simulink model "SimiSnake5"  (R2019a)
settings: Solver=VariableStepAuto  StartTime=0.0  StopTime=20  RelTol=1e-3  EnableMultiTasking=on
PreLoadFcn:
  | robotParameters;
undefined symbols (not defined in the file or in its folder): X, Y, Z
libraries: nesl_utility x49, sm_lib x38
(part 2 of 2)

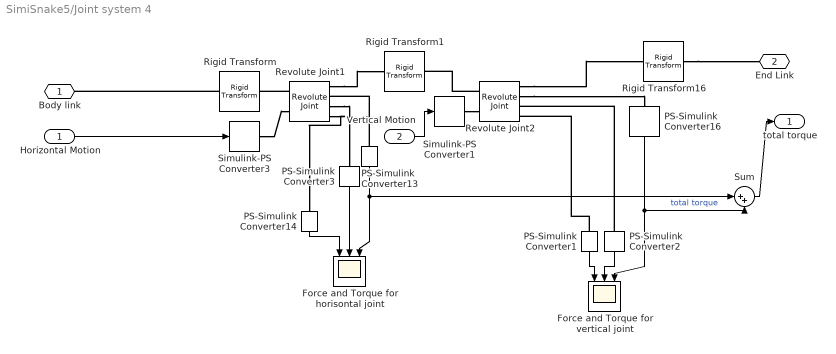
== system SimiSnake5/Joint system 4 ==
  Horizontal Motion : Inport
  Vertical Motion : Inport  Port=2
  Force and Torque for horisontal joint : Scope  NumInputPorts=3
  Force and Torque for vertical joint : Scope  NumInputPorts=3
  PS-Simulink Converter{1,13..14,16} (4 alike) : nesl_utility/PS-Simulink Converter  PhysicalDomain=network_engine_domain  SubClassName=ps_output  LeftPortType=input  RightPortType=output  PseudoPeriodic=off  Frequencies=[]  Unit=N*m  AffineConversion=off
  PS-Simulink Converter2 : nesl_utility/PS-Simulink Converter  PhysicalDomain=network_engine_domain  SubClassName=ps_output  LeftPortType=input  RightPortType=output  PseudoPeriodic=off  Frequencies=[]  Unit=N  AffineConversion=off
  PS-Simulink Converter3 : nesl_utility/PS-Simulink Converter  PhysicalDomain=network_engine_domain  SubClassName=ps_output  LeftPortType=input  RightPortType=output  PseudoPeriodic=off  Frequencies=[]  Unit=N  AffineConversion=off
  Revolute Joint1 : sm_lib/Joints/Revolute Joint  SenseConstraintForce=off  SenseConstraintForceX=off  SenseConstraintForceY=off  SenseConstraintForceZ=off  SenseConstraintTorque=off  SenseConstraintTorqueX=off  SenseConstraintTorqueY=off  SenseConstraintTorqueZ=off  SenseTotalForce=on  SenseTotalForceX=off  SenseTotalForceY=off  SenseTotalForceZ=off  SenseTotalTorque=on  SenseTotalTorqueX=off  SenseTotalTorqueY=off  SenseTotalTorqueZ=off  CompositeWrenchDir=FollowerOnBase  CompositeWrenchFrame=BaseFrame  EquilibriumPosition=0  EquilibriumPositionUnits=deg  SpringStiffness=0  SpringStiffnessUnits=N*m/deg  DampingCoefficient=0  DampingCoefficientUnits=N*m/(deg/s)  TorqueActuationMode=ComputedTorque  MotionActuationMode=InputMotion  SensePosition=off  SenseVelocity=off  SenseAcceleration=off  SenseTorqueForce=on  SenseLowerLimitTorqueForce=off  SenseUpperLimitTorqueForce=off  LowerLimitSpecify=off  LowerLimitBound=-90  LowerLimitBoundUnits=deg  LowerLimitStiffness=1e4  LowerLimitStiffnessUnits=N*m/deg  LowerLimitDamping=10  LowerLimitDampingUnits=N*m/(deg/s)  LowerLimitTransitionRegionWidth=0.1  LowerLimitTransitionRegionWidthUnits=deg  UpperLimitSpecify=off  UpperLimitBound=90  UpperLimitBoundUnits=deg  UpperLimitStiffness=1e4  UpperLimitStiffnessUnits=N*m/deg  UpperLimitDamping=10  UpperLimitDampingUnits=N*m/(deg/s)  UpperLimitTransitionRegionWidth=0.1  UpperLimitTransitionRegionWidthUnits=deg  PositionTargetSpecify=off  PositionTargetPriority=High  PositionTargetValue=30  PositionTargetValueUnits=deg  VelocityTargetSpecify=off  VelocityTargetPriority=High  VelocityTargetValue=0  VelocityTargetValueUnits=deg/s
  Revolute Joint2 : sm_lib/Joints/Revolute Joint  SenseConstraintForce=off  SenseConstraintForceX=off  SenseConstraintForceY=off  SenseConstraintForceZ=off  SenseConstraintTorque=off  SenseConstraintTorqueX=off  SenseConstraintTorqueY=off  SenseConstraintTorqueZ=off  SenseTotalForce=on  SenseTotalForceX=off  SenseTotalForceY=off  SenseTotalForceZ=off  SenseTotalTorque=on  SenseTotalTorqueX=off  SenseTotalTorqueY=off  SenseTotalTorqueZ=off  CompositeWrenchDir=FollowerOnBase  CompositeWrenchFrame=BaseFrame  EquilibriumPosition=0  EquilibriumPositionUnits=deg  SpringStiffness=0  SpringStiffnessUnits=N*m/deg  DampingCoefficient=0  DampingCoefficientUnits=N*m/(deg/s)  TorqueActuationMode=ComputedTorque  MotionActuationMode=InputMotion  SensePosition=off  SenseVelocity=off  SenseAcceleration=off  SenseTorqueForce=on  SenseLowerLimitTorqueForce=off  SenseUpperLimitTorqueForce=off  LowerLimitSpecify=off  LowerLimitBound=-90  LowerLimitBoundUnits=deg  LowerLimitStiffness=1e4  LowerLimitStiffnessUnits=N*m/deg  LowerLimitDamping=10  LowerLimitDampingUnits=N*m/(deg/s)  LowerLimitTransitionRegionWidth=0.1  LowerLimitTransitionRegionWidthUnits=deg  UpperLimitSpecify=off  UpperLimitBound=90  UpperLimitBoundUnits=deg  UpperLimitStiffness=1e4  UpperLimitStiffnessUnits=N*m/deg  UpperLimitDamping=10  UpperLimitDampingUnits=N*m/(deg/s)  UpperLimitTransitionRegionWidth=0.1  UpperLimitTransitionRegionWidthUnits=deg  PositionTargetSpecify=off  PositionTargetPriority=High  PositionTargetValue=30  PositionTargetValueUnits=deg  VelocityTargetSpecify=off  VelocityTargetPriority=High  VelocityTargetValue=0  VelocityTargetValueUnits=deg/s
  Rigid Transform : sm_lib/Frames and Transforms/Rigid Transform  TranslationMethod=StandardAxis  TranslationStandardOffset=5  TranslationLengthUnit=cm  TranslationStandardAxis=-Z  TranslationCartesianOffset=[0 0 0]  TranslationROffset=0  TranslationROffsetUnits=m  TranslationZOffset=0  TranslationZOffsetUnits=m  TranslationThetaOffset=0  TranslationThetaOffsetUnits=deg  RotationMethod=StandardAxis  RotationAngleUnits=deg  RotationStandardAxis=+X  RotationAngle=90  RotationArbitraryAxis=[0 0 1]  FollAlignAxisA=+X  BaseAlignAxisA=+Y  FollAlignAxisB=+Y  BaseAlignAxisB=+Z  RotationSequenceAxes=FollowerAxes  RotationSequence=XYX  RotationSequenceAngles=[0 0 0]  RotationSequenceAnglesUnits=deg  RotationMatrix=[1 0 0; 0 1 0; 0 0 1]
  Rigid Transform1 : sm_lib/Frames and Transforms/Rigid Transform  TranslationMethod=None  TranslationStandardOffset=5  TranslationLengthUnit=cm  TranslationStandardAxis=-Z  TranslationCartesianOffset=[0 0 0]  TranslationROffset=0  TranslationROffsetUnits=m  TranslationZOffset=0  TranslationZOffsetUnits=m  TranslationThetaOffset=0  TranslationThetaOffsetUnits=deg  RotationMethod=StandardAxis  RotationAngleUnits=deg  RotationStandardAxis=+X  RotationAngle=90  RotationArbitraryAxis=[0 0 1]  FollAlignAxisA=+X  BaseAlignAxisA=+Y  FollAlignAxisB=+Y  BaseAlignAxisB=+Z  RotationSequenceAxes=FollowerAxes  RotationSequence=XYX  RotationSequenceAngles=[0 0 0]  RotationSequenceAnglesUnits=deg  RotationMatrix=[1 0 0; 0 1 0; 0 0 1]
  Rigid Transform16 : sm_lib/Frames and Transforms/Rigid Transform  TranslationMethod=StandardAxis  TranslationStandardOffset=5  TranslationLengthUnit=cm  TranslationStandardAxis=+Z  TranslationCartesianOffset=[0 0 0]  TranslationROffset=0  TranslationROffsetUnits=m  TranslationZOffset=0  TranslationZOffsetUnits=m  TranslationThetaOffset=0  TranslationThetaOffsetUnits=deg  RotationMethod=StandardAxis  RotationAngleUnits=deg  RotationStandardAxis=-X  RotationAngle=180  RotationArbitraryAxis=[0 0 1]  FollAlignAxisA=+X  BaseAlignAxisA=+Y  FollAlignAxisB=+Y  BaseAlignAxisB=+Z  RotationSequenceAxes=FollowerAxes  RotationSequence=XYX  RotationSequenceAngles=[0 0 0]  RotationSequenceAnglesUnits=deg  RotationMatrix=[1 0 0; 0 1 0; 0 0 1]
  Simulink-PS Converter1 : nesl_utility/Simulink-PS Converter  PhysicalDomain=network_engine_domain  SubClassName=ps_input  LeftPortType=input  RightPortType=output  PseudoPeriodic=off  Frequencies=[]  NoiseDistribution=none  NoiseParameters=[]  Unit=deg  AffineConversion=off  FilteringAndDerivatives=filter  SimscapeFilterOrder=2  InputFilterTimeConstant=.01  UdotUserProvided=1
  Simulink-PS Converter3 : nesl_utility/Simulink-PS Converter  PhysicalDomain=network_engine_domain  SubClassName=ps_input  LeftPortType=input  RightPortType=output  PseudoPeriodic=off  Frequencies=[]  NoiseDistribution=none  NoiseParameters=[]  Unit=deg  AffineConversion=off  FilteringAndDerivatives=filter  SimscapeFilterOrder=2  InputFilterTimeConstant=.01  UdotUserProvided=1
  Sum : Sum  Inputs=|++
  Body link : PMIOPort  Side=Left
  "End Link " : PMIOPort  Port=2  Side=Right
  total torque : Outport
  wires:
  Vertical Motion/1 -> Simulink-PS Converter1/1
  PS-Simulink Converter14/1 -> Force and Torque for horisontal joint/1
  PS-Simulink Converter13/1 -> Force and Torque for horisontal joint/3, Sum/1
  PS-Simulink Converter3/1 -> Force and Torque for horisontal joint/2
  Horizontal Motion/1 -> Simulink-PS Converter3/1
  PS-Simulink Converter2/1 -> Force and Torque for vertical joint/2
  PS-Simulink Converter1/1 -> Force and Torque for vertical joint/1
  Sum/1 -> total torque/1
  PS-Simulink Converter16/1 -> Force and Torque for vertical joint/3, Sum/2  "total torque"
  connections:
  Simulink-PS Converter3/RConn1 -- Revolute Joint1/LConn2
  Revolute Joint1/RConn1 -- Rigid Transform1/LConn1
  Rigid Transform/LConn1 -- Body link/RConn1
  Revolute Joint1/RConn4 -- PS-Simulink Converter14/LConn1
  Revolute Joint1/RConn3 -- PS-Simulink Converter3/LConn1
  Revolute Joint2/RConn2 -- PS-Simulink Converter16/LConn1
  Revolute Joint2/RConn1 -- Rigid Transform16/LConn1
  PS-Simulink Converter13/LConn1 -- Revolute Joint1/RConn2
  Revolute Joint1/LConn1 -- Rigid Transform/RConn1
  Simulink-PS Converter1/RConn1 -- Revolute Joint2/LConn2
  Revolute Joint2/LConn1 -- Rigid Transform1/RConn1
  PS-Simulink Converter2/LConn1 -- Revolute Joint2/RConn3
  PS-Simulink Converter1/LConn1 -- Revolute Joint2/RConn4
  Rigid Transform16/RConn1 -- "End Link "/RConn1

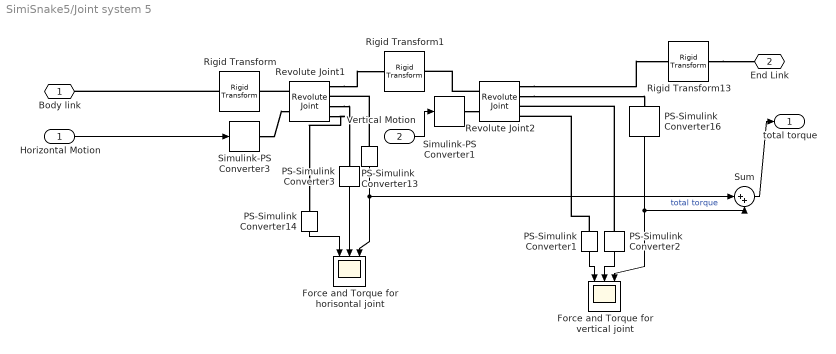
== system SimiSnake5/Joint system 5 ==
  Horizontal Motion : Inport
  Vertical Motion : Inport  Port=2
  Force and Torque for horisontal joint : Scope  NumInputPorts=3
  Force and Torque for vertical joint : Scope  NumInputPorts=3
  PS-Simulink Converter{1,13..14,16} (4 alike) : nesl_utility/PS-Simulink Converter  PhysicalDomain=network_engine_domain  SubClassName=ps_output  LeftPortType=input  RightPortType=output  PseudoPeriodic=off  Frequencies=[]  Unit=N*m  AffineConversion=off
  PS-Simulink Converter2 : nesl_utility/PS-Simulink Converter  PhysicalDomain=network_engine_domain  SubClassName=ps_output  LeftPortType=input  RightPortType=output  PseudoPeriodic=off  Frequencies=[]  Unit=N  AffineConversion=off
  PS-Simulink Converter3 : nesl_utility/PS-Simulink Converter  PhysicalDomain=network_engine_domain  SubClassName=ps_output  LeftPortType=input  RightPortType=output  PseudoPeriodic=off  Frequencies=[]  Unit=N  AffineConversion=off
  Revolute Joint1 : sm_lib/Joints/Revolute Joint  SenseConstraintForce=off  SenseConstraintForceX=off  SenseConstraintForceY=off  SenseConstraintForceZ=off  SenseConstraintTorque=off  SenseConstraintTorqueX=off  SenseConstraintTorqueY=off  SenseConstraintTorqueZ=off  SenseTotalForce=on  SenseTotalForceX=off  SenseTotalForceY=off  SenseTotalForceZ=off  SenseTotalTorque=on  SenseTotalTorqueX=off  SenseTotalTorqueY=off  SenseTotalTorqueZ=off  CompositeWrenchDir=FollowerOnBase  CompositeWrenchFrame=BaseFrame  EquilibriumPosition=0  EquilibriumPositionUnits=deg  SpringStiffness=0  SpringStiffnessUnits=N*m/deg  DampingCoefficient=0  DampingCoefficientUnits=N*m/(deg/s)  TorqueActuationMode=ComputedTorque  MotionActuationMode=InputMotion  SensePosition=off  SenseVelocity=off  SenseAcceleration=off  SenseTorqueForce=on  SenseLowerLimitTorqueForce=off  SenseUpperLimitTorqueForce=off  LowerLimitSpecify=off  LowerLimitBound=-90  LowerLimitBoundUnits=deg  LowerLimitStiffness=1e4  LowerLimitStiffnessUnits=N*m/deg  LowerLimitDamping=10  LowerLimitDampingUnits=N*m/(deg/s)  LowerLimitTransitionRegionWidth=0.1  LowerLimitTransitionRegionWidthUnits=deg  UpperLimitSpecify=off  UpperLimitBound=90  UpperLimitBoundUnits=deg  UpperLimitStiffness=1e4  UpperLimitStiffnessUnits=N*m/deg  UpperLimitDamping=10  UpperLimitDampingUnits=N*m/(deg/s)  UpperLimitTransitionRegionWidth=0.1  UpperLimitTransitionRegionWidthUnits=deg  PositionTargetSpecify=off  PositionTargetPriority=High  PositionTargetValue=30  PositionTargetValueUnits=deg  VelocityTargetSpecify=off  VelocityTargetPriority=High  VelocityTargetValue=0  VelocityTargetValueUnits=deg/s
  Revolute Joint2 : sm_lib/Joints/Revolute Joint  SenseConstraintForce=off  SenseConstraintForceX=off  SenseConstraintForceY=off  SenseConstraintForceZ=off  SenseConstraintTorque=off  SenseConstraintTorqueX=off  SenseConstraintTorqueY=off  SenseConstraintTorqueZ=off  SenseTotalForce=on  SenseTotalForceX=off  SenseTotalForceY=off  SenseTotalForceZ=off  SenseTotalTorque=on  SenseTotalTorqueX=off  SenseTotalTorqueY=off  SenseTotalTorqueZ=off  CompositeWrenchDir=FollowerOnBase  CompositeWrenchFrame=BaseFrame  EquilibriumPosition=0  EquilibriumPositionUnits=deg  SpringStiffness=0  SpringStiffnessUnits=N*m/deg  DampingCoefficient=0  DampingCoefficientUnits=N*m/(deg/s)  TorqueActuationMode=ComputedTorque  MotionActuationMode=InputMotion  SensePosition=off  SenseVelocity=off  SenseAcceleration=off  SenseTorqueForce=on  SenseLowerLimitTorqueForce=off  SenseUpperLimitTorqueForce=off  LowerLimitSpecify=off  LowerLimitBound=-90  LowerLimitBoundUnits=deg  LowerLimitStiffness=1e4  LowerLimitStiffnessUnits=N*m/deg  LowerLimitDamping=10  LowerLimitDampingUnits=N*m/(deg/s)  LowerLimitTransitionRegionWidth=0.1  LowerLimitTransitionRegionWidthUnits=deg  UpperLimitSpecify=off  UpperLimitBound=90  UpperLimitBoundUnits=deg  UpperLimitStiffness=1e4  UpperLimitStiffnessUnits=N*m/deg  UpperLimitDamping=10  UpperLimitDampingUnits=N*m/(deg/s)  UpperLimitTransitionRegionWidth=0.1  UpperLimitTransitionRegionWidthUnits=deg  PositionTargetSpecify=off  PositionTargetPriority=High  PositionTargetValue=30  PositionTargetValueUnits=deg  VelocityTargetSpecify=off  VelocityTargetPriority=High  VelocityTargetValue=0  VelocityTargetValueUnits=deg/s
  Rigid Transform : sm_lib/Frames and Transforms/Rigid Transform  TranslationMethod=StandardAxis  TranslationStandardOffset=5  TranslationLengthUnit=cm  TranslationStandardAxis=-Z  TranslationCartesianOffset=[0 0 0]  TranslationROffset=0  TranslationROffsetUnits=m  TranslationZOffset=0  TranslationZOffsetUnits=m  TranslationThetaOffset=0  TranslationThetaOffsetUnits=deg  RotationMethod=StandardAxis  RotationAngleUnits=deg  RotationStandardAxis=+X  RotationAngle=90  RotationArbitraryAxis=[0 0 1]  FollAlignAxisA=+X  BaseAlignAxisA=+Y  FollAlignAxisB=+Y  BaseAlignAxisB=+Z  RotationSequenceAxes=FollowerAxes  RotationSequence=XYX  RotationSequenceAngles=[0 0 0]  RotationSequenceAnglesUnits=deg  RotationMatrix=[1 0 0; 0 1 0; 0 0 1]
  Rigid Transform1 : sm_lib/Frames and Transforms/Rigid Transform  TranslationMethod=None  TranslationStandardOffset=5  TranslationLengthUnit=cm  TranslationStandardAxis=-Z  TranslationCartesianOffset=[0 0 0]  TranslationROffset=0  TranslationROffsetUnits=m  TranslationZOffset=0  TranslationZOffsetUnits=m  TranslationThetaOffset=0  TranslationThetaOffsetUnits=deg  RotationMethod=StandardAxis  RotationAngleUnits=deg  RotationStandardAxis=+X  RotationAngle=90  RotationArbitraryAxis=[0 0 1]  FollAlignAxisA=+X  BaseAlignAxisA=+Y  FollAlignAxisB=+Y  BaseAlignAxisB=+Z  RotationSequenceAxes=FollowerAxes  RotationSequence=XYX  RotationSequenceAngles=[0 0 0]  RotationSequenceAnglesUnits=deg  RotationMatrix=[1 0 0; 0 1 0; 0 0 1]
  Rigid Transform13 : sm_lib/Frames and Transforms/Rigid Transform  TranslationMethod=StandardAxis  TranslationStandardOffset=5  TranslationLengthUnit=cm  TranslationStandardAxis=+Z  TranslationCartesianOffset=[0 0 0]  TranslationROffset=0  TranslationROffsetUnits=m  TranslationZOffset=0  TranslationZOffsetUnits=m  TranslationThetaOffset=0  TranslationThetaOffsetUnits=deg  RotationMethod=StandardAxis  RotationAngleUnits=deg  RotationStandardAxis=-X  RotationAngle=180  RotationArbitraryAxis=[0 0 1]  FollAlignAxisA=+X  BaseAlignAxisA=+Y  FollAlignAxisB=+Y  BaseAlignAxisB=+Z  RotationSequenceAxes=FollowerAxes  RotationSequence=XYX  RotationSequenceAngles=[0 0 0]  RotationSequenceAnglesUnits=deg  RotationMatrix=[1 0 0; 0 1 0; 0 0 1]
  Simulink-PS Converter1 : nesl_utility/Simulink-PS Converter  PhysicalDomain=network_engine_domain  SubClassName=ps_input  LeftPortType=input  RightPortType=output  PseudoPeriodic=off  Frequencies=[]  NoiseDistribution=none  NoiseParameters=[]  Unit=deg  AffineConversion=off  FilteringAndDerivatives=filter  SimscapeFilterOrder=2  InputFilterTimeConstant=.01  UdotUserProvided=1
  Simulink-PS Converter3 : nesl_utility/Simulink-PS Converter  PhysicalDomain=network_engine_domain  SubClassName=ps_input  LeftPortType=input  RightPortType=output  PseudoPeriodic=off  Frequencies=[]  NoiseDistribution=none  NoiseParameters=[]  Unit=deg  AffineConversion=off  FilteringAndDerivatives=filter  SimscapeFilterOrder=2  InputFilterTimeConstant=.01  UdotUserProvided=1
  Sum : Sum  Inputs=|++
  Body link : PMIOPort  Side=Left
  "End Link " : PMIOPort  Port=2  Side=Right
  total torque : Outport
  wires:
  Vertical Motion/1 -> Simulink-PS Converter1/1
  PS-Simulink Converter14/1 -> Force and Torque for horisontal joint/1
  PS-Simulink Converter13/1 -> Force and Torque for horisontal joint/3, Sum/1
  PS-Simulink Converter3/1 -> Force and Torque for horisontal joint/2
  Horizontal Motion/1 -> Simulink-PS Converter3/1
  PS-Simulink Converter2/1 -> Force and Torque for vertical joint/2
  PS-Simulink Converter1/1 -> Force and Torque for vertical joint/1
  Sum/1 -> total torque/1
  PS-Simulink Converter16/1 -> Force and Torque for vertical joint/3, Sum/2  "total torque"
  connections:
  Simulink-PS Converter3/RConn1 -- Revolute Joint1/LConn2
  Revolute Joint1/RConn1 -- Rigid Transform1/LConn1
  Rigid Transform/LConn1 -- Body link/RConn1
  Revolute Joint1/RConn4 -- PS-Simulink Converter14/LConn1
  Revolute Joint1/RConn3 -- PS-Simulink Converter3/LConn1
  Revolute Joint2/RConn2 -- PS-Simulink Converter16/LConn1
  Rigid Transform13/RConn1 -- "End Link "/RConn1
  PS-Simulink Converter13/LConn1 -- Revolute Joint1/RConn2
  Revolute Joint1/LConn1 -- Rigid Transform/RConn1
  Simulink-PS Converter1/RConn1 -- Revolute Joint2/LConn2
  Revolute Joint2/LConn1 -- Rigid Transform1/RConn1
  PS-Simulink Converter2/LConn1 -- Revolute Joint2/RConn3
  PS-Simulink Converter1/LConn1 -- Revolute Joint2/RConn4
  Revolute Joint2/RConn1 -- Rigid Transform13/LConn1

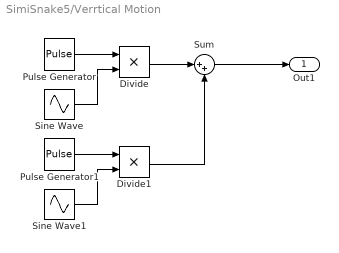
== system SimiSnake5/Verrtical Motion  ==
  Divide : Product  Inputs=**
  Divide1 : Product  Inputs=**
  Pulse Generator : DiscretePulseGenerator  PulseType=Time based  PulseWidth=50
  Pulse Generator1 : DiscretePulseGenerator  PulseType=Time based  PulseWidth=50  PhaseDelay=1
  Sine Wave : Sin  Amplitude=20  Frequency=5  Phase=2.09
  Sine Wave1 : Sin  Amplitude=15  Frequency=5  Phase=2.09
  Sum : Sum  Inputs=|++
  Out1 : Outport
  wires:
  Sum/1 -> Out1/1
  Divide1/1 -> Sum/2
  Divide/1 -> Sum/1
  Pulse Generator/1 -> Divide/1
  Sine Wave1/1 -> Divide1/2
  Sine Wave/1 -> Divide/2
  Pulse Generator1/1 -> Divide1/1

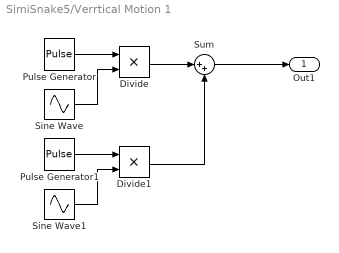
== system SimiSnake5/Verrtical Motion 1 ==
  Divide : Product  Inputs=**
  Divide1 : Product  Inputs=**
  Pulse Generator : DiscretePulseGenerator  PulseType=Time based  PulseWidth=50
  Pulse Generator1 : DiscretePulseGenerator  PulseType=Time based  PulseWidth=50  PhaseDelay=1
  Sine Wave : Sin  Amplitude=20  Frequency=5  Phase=2 * 2.09  SampleTime=0
  Sine Wave1 : Sin  Amplitude=15  Frequency=5  Phase=2.09 * 2  SampleTime=0
  Sum : Sum  Inputs=|++
  Out1 : Outport
  wires:
  Sum/1 -> Out1/1
  Divide1/1 -> Sum/2
  Divide/1 -> Sum/1
  Pulse Generator/1 -> Divide/1
  Sine Wave1/1 -> Divide1/2
  Sine Wave/1 -> Divide/2
  Pulse Generator1/1 -> Divide1/1

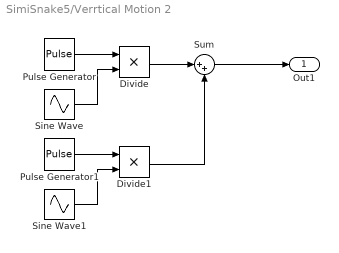
== system SimiSnake5/Verrtical Motion 2 ==
  Divide : Product  Inputs=**
  Divide1 : Product  Inputs=**
  Pulse Generator : DiscretePulseGenerator  PulseType=Time based  PulseWidth=50
  Pulse Generator1 : DiscretePulseGenerator  PulseType=Time based  PulseWidth=50  PhaseDelay=1
  Sine Wave : Sin  Amplitude=20  Frequency=5  Phase=2.09 * 3  SampleTime=0
  Sine Wave1 : Sin  Amplitude=15  Frequency=5  Phase=2.09 * 3  SampleTime=0
  Sum : Sum  Inputs=|++
  Out1 : Outport
  wires:
  Sum/1 -> Out1/1
  Divide1/1 -> Sum/2
  Divide/1 -> Sum/1
  Pulse Generator/1 -> Divide/1
  Sine Wave1/1 -> Divide1/2
  Sine Wave/1 -> Divide/2
  Pulse Generator1/1 -> Divide1/1

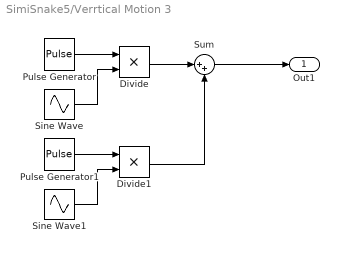
== system SimiSnake5/Verrtical Motion 3 ==
  Divide : Product  Inputs=**
  Divide1 : Product  Inputs=**
  Pulse Generator : DiscretePulseGenerator  PulseType=Time based  PulseWidth=50
  Pulse Generator1 : DiscretePulseGenerator  PulseType=Time based  PulseWidth=50  PhaseDelay=1
  Sine Wave : Sin  Amplitude=20  Frequency=5  Phase=2.09 * 4  SampleTime=0
  Sine Wave1 : Sin  Amplitude=15  Frequency=5  Phase=2.09 * 4  SampleTime=0
  Sum : Sum  Inputs=|++
  Out1 : Outport
  wires:
  Sum/1 -> Out1/1
  Divide1/1 -> Sum/2
  Divide/1 -> Sum/1
  Pulse Generator/1 -> Divide/1
  Sine Wave1/1 -> Divide1/2
  Sine Wave/1 -> Divide/2
  Pulse Generator1/1 -> Divide1/1

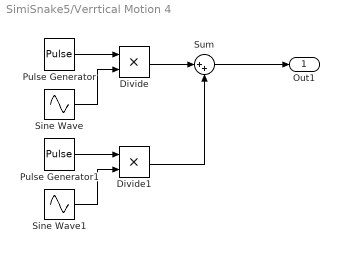
== system SimiSnake5/Verrtical Motion 4 ==
  Divide : Product  Inputs=**
  Divide1 : Product  Inputs=**
  Pulse Generator : DiscretePulseGenerator  PulseType=Time based  PulseWidth=50
  Pulse Generator1 : DiscretePulseGenerator  PulseType=Time based  PulseWidth=50  PhaseDelay=1
  Sine Wave : Sin  Amplitude=20  Frequency=5  Phase=2.09 * 5  SampleTime=0
  Sine Wave1 : Sin  Amplitude=15  Frequency=5  Phase=2.09 * 5  SampleTime=0
  Sum : Sum  Inputs=|++
  Out1 : Outport
  wires:
  Sum/1 -> Out1/1
  Divide1/1 -> Sum/2
  Divide/1 -> Sum/1
  Pulse Generator/1 -> Divide/1
  Sine Wave1/1 -> Divide1/2
  Sine Wave/1 -> Divide/2
  Pulse Generator1/1 -> Divide1/1

== system SimiSnake5/Verrtical Motion 5 ==
  Divide : Product  Inputs=**
  Divide1 : Product  Inputs=**
  Pulse Generator : DiscretePulseGenerator  PulseType=Time based  PulseWidth=50
  Pulse Generator1 : DiscretePulseGenerator  PulseType=Time based  PulseWidth=50  PhaseDelay=1
  Sine Wave : Sin  Amplitude=20  Frequency=5  Phase=2.09 * 6  SampleTime=0
  Sine Wave1 : Sin  Amplitude=15  Frequency=5  Phase=2.09 * 6  SampleTime=0
  Sum : Sum  Inputs=|++
  Out1 : Outport
  wires:
  Sum/1 -> Out1/1
  Divide1/1 -> Sum/2
  Divide/1 -> Sum/1
  Pulse Generator/1 -> Divide/1
  Sine Wave1/1 -> Divide1/2
  Sine Wave/1 -> Divide/2
  Pulse Generator1/1 -> Divide1/1
